simulink model "untitled"  (R2015b)
settings: Solver=ode45  StartTime=0.0  StopTime=10  RelTol=1e-6
undefined symbols (not defined in the file or in its folder): magnitude
libraries: simulink x4
settings Model: Creator=JohnYang  LastModifiedBy=Yang Yang
settings DataIOCC: SaveFormat=Array
settings HardwareCC: ProdBitPerPointer=32  ProdLargestAtomicFloat=None  ProdIntDivRoundTo=Undefined  ProdEndianess=Unspecified  ProdWordSize=32  ProdHWDeviceType=32-bit Generic
settings GRTTargetCC: GeneratePreprocessorConditionals=Disable all
settings ConfigComp: CovModelRefEnable=Off

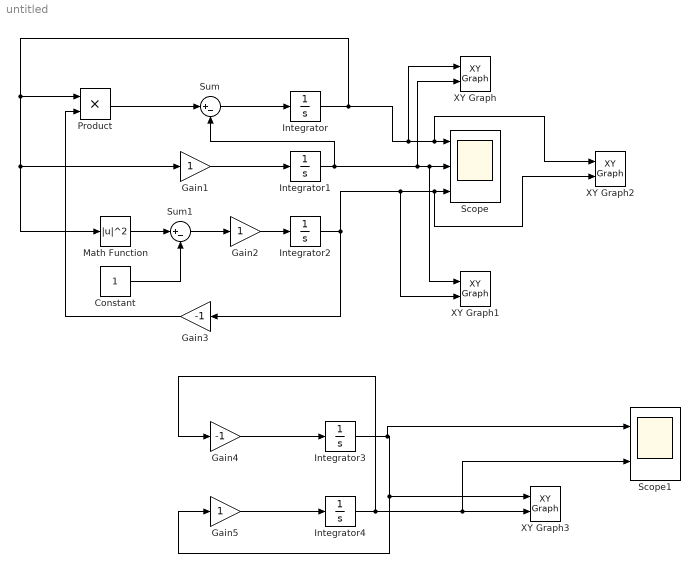
== system untitled ==
  Constant : Constant
  Gain1 : Gain
  Gain2 : Gain
  Gain3 : Gain  Gain=-1
  Gain4 : Gain  Gain=-1
  Gain5 : Gain
  Integrator{,1..4} (5 alike) : Integrator
  Math Function : Math  Operator=magnitude^2  SaturateOnIntegerOverflow=on
  Product : Product
  Scope : Scope  NumInputPorts=3
  Scope1 : Scope  NumInputPorts=2
  Sum : Sum  Inputs=|+-
  Sum1 : Sum  Inputs=|+-
  XY Graph{,1..3} (4 alike) : simulink/Sinks/XY Graph  xmin=-1  xmax=1  ymin=-1  ymax=1  st=-1
  wires:
  Gain3/1 -> Product/2
  Product/1 -> Sum/1
  Sum/1 -> Integrator/1
  Integrator1/1 -> Scope/2, XY Graph1/1, XY Graph/2, Sum/2
  Gain1/1 -> Integrator1/1
  Gain2/1 -> Integrator2/1
  Sum1/1 -> Gain2/1
  Math Function/1 -> Sum1/1
  Constant/1 -> Sum1/2
  Integrator2/1 -> Gain3/1, XY Graph2/2, Scope/3, XY Graph1/2
  Integrator/1 -> Product/1, Gain1/1, Math Function/1, XY Graph/1, XY Graph2/1, Scope/1
  Gain4/1 -> Integrator3/1
  Gain5/1 -> Integrator4/1
  Integrator4/1 -> Scope1/2, XY Graph3/2, Gain4/1
  Integrator3/1 -> Scope1/1, Gain5/1, XY Graph3/1
